simulink model "W3_prob2"  (R2020b)
settings: Solver=VariableStepAuto  StartTime=0.0  StopTime=inf  RelTol=1e-3
settings Model: Creator=user  LastModifiedBy=user

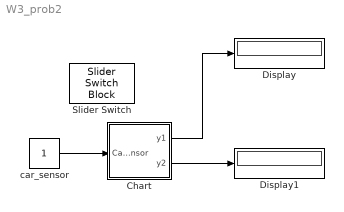
== system W3_prob2 ==
  Chart : Stateflow chart  TreatAsAtomicUnit=on
  Display : Display
  Display1 : Display
  Slider Switch : SliderSwitchBlock  LabelPosition=Hide
      settings: Values={{'Off', 'On'}, [0 1]}
  car_sensor : Constant
  wires:
  Chart/1(y1) -> Display/1
  Chart/2(y2) -> Display1/1
  car_sensor/1 -> Chart/1(Car_Sensor)

== stateflow chart W3_prob2/Chart ==
  state Stop
    en:y1=Red;
    y2=Green;
  state StopForTraffic
    en:
    y1=Red;
    y2=Green;
  state StopToGo
    en:
    y1=Red;
    y2=Yellow;
  state GoToStop
    en:
    y1=Yellow;
    y2=Red;
  state Go
    en:
    y1=Green;
    y2=Red;
  (default) -> Stop
  Stop -> StopForTraffic : after(20,sec)
  StopForTraffic -> StopToGo : [Car_Sensor]
  GoToStop -> Stop : after(3,sec)
  StopToGo -> Go : after(3,sec)
  Go -> GoToStop : after(10,sec)
  data: Green constant double =3; Yellow constant double =2; Red constant double =1; y1 output; Car_Sensor input; y2 output
